simulink model "SST_FINAL_SIMULINK"  (R2017b)
settings: Solver=ode14x  StartTime=0.0  StopTime=120/60  MaxStep=1e-4  RelTol=1e-3
values from neighbouring files (symbols this model uses):
  C_3P4L = (Potencia_nominal)/(2*pi*60*0.1*((Entrada)^2))    (= 0.00858724363662)    [SST_FINAL.m]
  C_HB = 50000/(0.6*60*pi*(11397^2))    (= 3.40358447746e-06)    [SST_FINAL.m]
  ca = 1/(L*a)    [SST_FINAL.m]
  CDAB1 = 50*(Pnom/3)/(Vmin_DAB1^2*Fsw_DAB)    [SST_FINAL.m]
  CDAB2 = 50*(Pnom/3)/(Vmin_DAB2^2*Fsw_DAB)    [SST_FINAL.m]
  E = Nm*Vout_HB    (= 11397)    [SST_FINAL.m]
  Fsw_DAB = 30e3    (= 30000)    [SST_FINAL.m]
  Fsw_HB = 15e3    (= 15000)    [SST_FINAL.m]
  Fsw_NPC = 5040    [SST_FINAL.m]
  Inom_HB = (50e3/(13200*sqrt(3)))*sqrt(2)    [SST_FINAL.m]
  Kc_I = H_infI    [SST_FINAL.m]
  Kc_V = H_infV    [SST_FINAL.m]
  KcI_DAB = H_infI_DAB    [SST_FINAL.m]
  KcV_DAB = H_infV_DAB    [SST_FINAL.m]
  Ki = 2.5641    [SST_FINAL.m]
  Kp = 0.00138    [SST_FINAL.m]
  L = ((0.03*Entrada))/((2*pi*60)*(Imax))    [SST_FINAL.m]
  L_DAB = (1/Ntr)*VDAB1*VDAB2*D*(1-D)/(2*Fsw_DAB*(Pnom/3))    (= 2.89591875e-05)    [SST_FINAL.m]
  L_HB = 50e-3    (= 0.05)    [SST_FINAL.m]
  m = (2*Voltaje_pico)/Entrada    [SST_FINAL.m]
  Pnom = 50e3    (= 50000)    [SST_FINAL.m]
  R_DAB = 30e3*2*pi*L_DAB*0.1    (= 0.545867824224)    [SST_FINAL.m]
  R_HB = 120*pi*L_HB*0.05    (= 0.942477796077)    [SST_FINAL.m]
  R_LOAD2 = VDAB2^2/(Pnom/3)    (= 9.26694)    [SST_FINAL.m]
  tauI_I = 1/(2*pi*F_lagI)    (= 0.00265258238486)    [SST_FINAL.m]
  tauI_V = 1/(2*pi*F_LagV)    (= 0.00039788735773)    [SST_FINAL.m]
  tauII_DAB = 1/(2*pi*F_lagI_DAB)    (= 0.00265258238486)    [SST_FINAL.m]
  tauIV_DAB = 1/(2*pi*F_lagV_DAB)    (= 0.265258238486)    [SST_FINAL.m]
  Ts = 1/(200*Fsw_DAB)    (= 1.66666666667e-07)    [SST_FINAL.m]
  uLmt_dDAB = 0.5    [SST_FINAL.m]
  uLmt_I = 0.05    [SST_FINAL.m]
  uLmt_V = Inom_HB    [SST_FINAL.m]
  VDAB1 = 11397    [SST_FINAL.m]
  VDAB2 = 393    [SST_FINAL.m]
  Vp = Entrada/2    (= 196.5)    [SST_FINAL.m]
  W = 120*pi    (= 376.991118431)    [SST_FINAL.m]
  w = 120*pi    (= 376.991118431)    [SST_FINAL.m]
libraries: powerlib x102, powerlib_meascontrol x26, simulink x16, dspstat3 x3
(part 1 of 2)
settings Model: SimulationMode=accelerator  Creator=Sergio  LastModifiedBy=Sergio

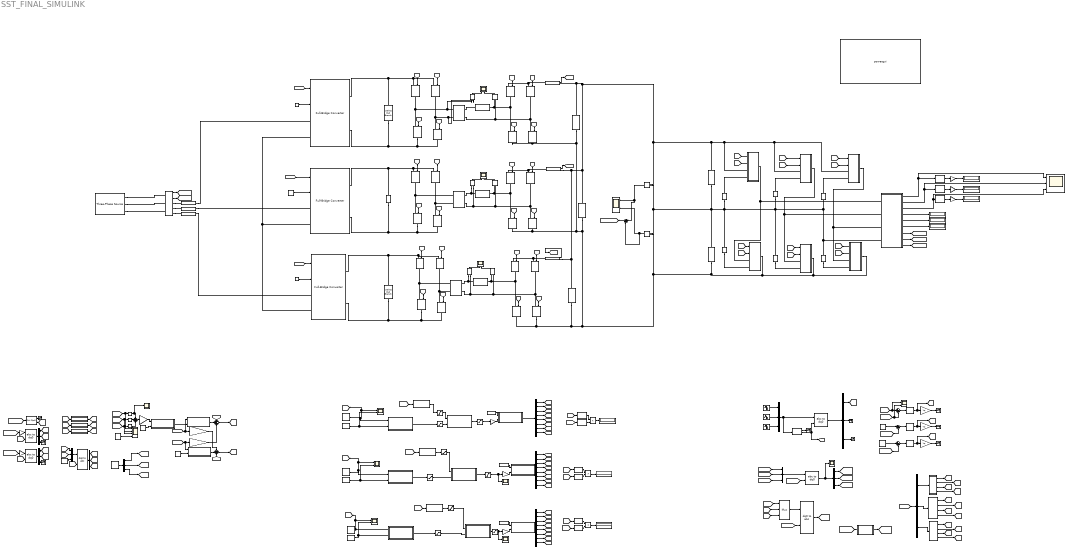
== system SST_FINAL_SIMULINK ==
  note: Fuente Trifásica Balanceada
      | Sec(+) Vnom=13.2 [kV]
  note: Medición de tensión y corriente
      | en media tensión
  note: Lazo de control de corriente
      | para etapa rectificadora
  note: Lazo de control de tensión
      | para etapa rectificadora
  note: Conversión de referencia abc a dq0
  note: Generación de pulsos - Metodo SPWM
  note: Conversión de referencia dq0 a abc
  note: Transformador Trifásico de Estado Sólido de Flujo Unidireccional de tres etapas de 13.2KV a 220V
  note: CONTROLADOR Y MODULADOR ETAPA AC-DC
  note: CONTROLADOR Y MODULADOR ETAPA DC-DC
  note: MODULADOR PSM
  note: MODULADOR PSM
  note: MODULADOR PSM
  note: CONTROLADOR LAZO
      | DE CORRIENTE
  note: CONTROLADOR LAZO
      | DE CORRIENTE
  note: CONTROLADOR LAZO
      | DE CORRIENTE
  note: CONTROLADOR LAZO
      | DE TENSIÓN
  note: CONTROLADOR LAZO
      | DE TENSIÓN
  note: CONTROLADOR LAZO
      | DE TENSIÓN
  note: POTENCIA DAB1
  note: POTENCIA DAB2
  note: POTENCIA DAB3
  note: CONTROLADOR Y MODULADOR ETAPA DC-AC
  note: ETAPA AC-DC
  note: ETAPA DC-DC
  note: ETAPA DC-AC
  note: CARGA CONECTADA EN Y
  note: TENSIONES DE LINEA EN LA CARGA
  note: TENSIONES RMS DE LINEA EN LA CARGA
  note: THD VAB
  note: THD VBC
  note: THD VCA
  note: TENSIONES CHB
  note: TENSIONES CHB
      | AVERAGE
  note: TENSIÓN VDAB2
  note: TENSIÓN VDAB2
  note: TENSIÓN VDAB2
  note: TENSIONES FASE DE REFERENCIA EN DQ0
  note: TENSIONES FASE MEDIDAS EN DQ0
  note: BALANCEO DE LAS CAPACITANCIAS NPC
  note: CONTROLADOR DE TENSIÓN EN EL DOMINIO DQ0
  note: CONVERSIÓN DE DQ0 A ABC DE LOS PULSOS
  note: GENERACIÓN DE PULSOS METODO SPWM
  note: TENSIÓN CAPACITANCIAS NPC
  CONTROL_ID_buck2 : MATLAB Function  TreatAsAtomicUnit=on
  CONTROL_ID_buck3 : MATLAB Function  TreatAsAtomicUnit=on
  CONTROL_ID_buck5 : MATLAB Function  TreatAsAtomicUnit=on
  CONTROL_ID_buck6 : MATLAB Function  TreatAsAtomicUnit=on
  CONTROL_ID_buck8 : MATLAB Function  TreatAsAtomicUnit=on
  CONTROL_ID_buck9 : MATLAB Function  TreatAsAtomicUnit=on
  Carga R con Filtro LC : Subsystem
  Constant : Constant  Value=VDAB2  SampleTime=Ts
  Constant{3..5,10,12,19..20} (7 alike) : Constant  Value=0
  Constant11 : Constant
  Constant8 : Constant  Value=VDAB2  SampleTime=Ts
  Constant9 : Constant  Value=VDAB2  SampleTime=Ts
  Current Measurement1 : powerlib/Measurements/Current Measurement  PhasorSimulation=off  OutputType=Complex  PSBequivalent=0
  Current Measurement2 : powerlib/Measurements/Current Measurement  PhasorSimulation=off  OutputType=Complex  PSBequivalent=0
  Current Measurement3 : powerlib/Measurements/Current Measurement  PhasorSimulation=off  OutputType=Complex  PSBequivalent=0
  D{1..5,7} (6 alike) : powerlib/Power Electronics/Diode  Ron=0.001  Lon=0  Vf=0  IC=0  UseSnubber=off  Rs=500  Cs=250e-9  Measurements=off
  DAB1_S{1..24} (24 alike) : powerlib/Power Electronics/IGBT//Diode  Ron=1e-3  Rs=1e5  Cs=inf  Measurements=off
  Demux : Demux  Outputs=8
  Demux1 : Demux  Outputs=8
  Demux{7..13} (7 alike) : Demux  Outputs=3
  Demux2 : Demux  Outputs=8
  Display{2..4,7..12} (9 alike) : Display
  Fase A1 : Sin  Amplitude=(220*sqrt(2))/sqrt(3)  Frequency=120*pi  SampleTime=0
  Fase B1 : Sin  Amplitude=(220*sqrt(2))/sqrt(3)  Frequency=120*pi  Phase=-120*pi/180  SampleTime=0
  Fase C1 : Sin  Amplitude=(220*sqrt(2))/sqrt(3)  Frequency=120*pi  Phase=120*pi/180  SampleTime=0
  Gain10 : Gain  Gain=100
  Gain11 : Gain  Gain=Vp
  Gain12 : Gain  Gain=Vp
  Gain13 : Gain  Gain=Vp
  Gain14 : Gain  Gain=1/E
  Gain15 : Gain  Gain=1/Inom_HB
  Gain16 : Gain  Gain=1/(3*E)
  Gain17 : Gain  Gain=W*L_HB*Inom_HB/E
  Gain18 : Gain  Gain=W*L_HB*Inom_HB/E
  Gain2 : Gain  Gain=pi
  Gain3 : Gain  Gain=100
  Gain4 : Gain  Gain=pi
  Gain5 : Gain  Gain=pi
  Gain8 : Gain  Gain=100
  H-Bridge A : powerlib/Power Electronics/Full-Bridge Converter  ModelType=Switching devices  Ron=1e-3  Rs=1e6  Cs=inf  Vforward=[0,0]  Ron_Diode=1e-3  Rs_Diode=1e6  Cs_Diode=inf  Vf_Diode=1e-3  Rs_CurrentSource=inf
      settings: SourceProductName=Simscape Power Systems  SourceProductBaseCode=PS
  H-Bridge B : powerlib/Power Electronics/Full-Bridge Converter  ModelType=Switching devices  Ron=1e-3  Rs=1e6  Cs=inf  Vforward=[0,0]  Ron_Diode=1e-3  Rs_Diode=1e6  Cs_Diode=inf  Vf_Diode=1e-3  Rs_CurrentSource=inf
      settings: SourceProductName=Simscape Power Systems  SourceProductBaseCode=PS
  H-Bridge C : powerlib/Power Electronics/Full-Bridge Converter  ModelType=Switching devices  Ron=1e-3  Rs=1e6  Cs=inf  Vforward=[0,0]  Ron_Diode=1e-3  Rs_Diode=1e6  Cs_Diode=inf  Vf_Diode=1e-3  Rs_CurrentSource=inf
      settings: SourceProductName=Simscape Power Systems  SourceProductBaseCode=PS
  LA : powerlib/Elements/Series RLC Branch  LConnTagsString=__new0  RConnTagsString=__new0  BranchType=RL  Resistance=R_HB  Inductance=L_HB  SetiL0=off  InitialCurrent=Inom  Capacitance=1e-6  Setx0=off  InitialVoltage=0  Measurements=None
  LB : powerlib/Elements/Series RLC Branch  LConnTagsString=__new0  RConnTagsString=__new0  BranchType=RL  Resistance=R_HB  Inductance=L_HB  SetiL0=off  InitialCurrent=Inom  Capacitance=1e-6  Setx0=off  InitialVoltage=0  Measurements=None
  LC : powerlib/Elements/Series RLC Branch  LConnTagsString=__new0  RConnTagsString=__new0  BranchType=RL  Resistance=R_HB  Inductance=L_HB  SetiL0=off  InitialCurrent=Inom  Capacitance=1e-6  Setx0=off  InitialVoltage=0  Measurements=None
  Linear Transformer1 : powerlib/Elements/Linear Transformer  UNITS=pu  NominalPower=[Pnom Fsw_DAB]  winding1=[VDAB1 0 0]  winding2=[VDAB2 0 0]  ThreeWindings=off  winding3=[ 315e3 0.002 0.08 ]  RmLm=[100e6 inf]  Measurements=None  DataType=off
  Linear Transformer2 : powerlib/Elements/Linear Transformer  UNITS=pu  NominalPower=[Pnom Fsw_DAB]  winding1=[VDAB1 0 0]  winding2=[VDAB2 0 0]  ThreeWindings=off  winding3=[ 315e3 0.002 0.08 ]  RmLm=[100e6 inf]  Measurements=None  DataType=off
  Linear Transformer3 : powerlib/Elements/Linear Transformer  UNITS=pu  NominalPower=[Pnom Fsw_DAB]  winding1=[VDAB1 0 0]  winding2=[VDAB2 0 0]  ThreeWindings=off  winding3=[ 315e3 0.002 0.08 ]  RmLm=[100e6 inf]  Measurements=None  DataType=off
  MATLAB Function2 : MATLAB Function  TreatAsAtomicUnit=on
  MATLAB Function3 : MATLAB Function  TreatAsAtomicUnit=on
  MATLAB Function4 : MATLAB Function  TreatAsAtomicUnit=on
  MATLAB Function5 : MATLAB Function  TreatAsAtomicUnit=on
  MATLAB Function6 : MATLAB Function  TreatAsAtomicUnit=on
  MATLAB Function7 : MATLAB Function  TreatAsAtomicUnit=on
  Mean{,1..5} (6 alike) : powerlib_meascontrol/Measurements/Mean  Freq=Fsw_DAB  Vinit=0  Ts=Ts
  Mean6 : powerlib_meascontrol/Measurements/Mean  Freq=120  Vinit=0  Ts=Ts
  Mean7 : powerlib_meascontrol/Measurements/Mean  Freq=120  Vinit=0  Ts=Ts
  Mean8 : powerlib_meascontrol/Measurements/Mean  Freq=120  Vinit=0  Ts=Ts
  Moving Average : dspstat3/Moving Average  Method=Sliding window  SpecifyWindowLength=on  WindowLength=1000  ForgettingFactor=0.9  SimulateUsing=Code generation
  Moving Average1 : dspstat3/Moving Average  Method=Sliding window  SpecifyWindowLength=on  WindowLength=1000  ForgettingFactor=0.9  SimulateUsing=Code generation
  Moving Average2 : dspstat3/Moving Average  Method=Sliding window  SpecifyWindowLength=on  WindowLength=1000  ForgettingFactor=0.9  SimulateUsing=Code generation
  Multimeter : powerlib/Measurements/Multimeter  PhasorSimulation=off  OutputType=Complex  sel=3  L=6  Gain=1  yselected={'Ub: Series RLC Branch16'};  PSBOutputType=1  PSBequivalent=0  AxesSetting=[0,0.1,-100,100]  Display=0  SavedBlockNames=-11
  Multimeter1 : powerlib/Measurements/Multimeter  PhasorSimulation=off  OutputType=Complex  sel=1  L=6  Gain=1  yselected={'Ub: Series RLC Branch13'};  PSBOutputType=1  PSBequivalent=0  AxesSetting=[0,0.1,-100,100]  Display=0  SavedBlockNames=-11
  Multimeter2 : powerlib/Measurements/Multimeter  PhasorSimulation=off  OutputType=Complex  sel=2  L=6  Gain=1  yselected={'Ub: Series RLC Branch14'};  PSBOutputType=1  PSBequivalent=0  AxesSetting=[0,0.1,-100,100]  Display=0  SavedBlockNames=-11
  Multimeter4 : powerlib/Measurements/Multimeter  PhasorSimulation=off  OutputType=Complex  sel=[4 5 6]  L=6  Gain=[1 1 1]  yselected={'Ub: Vout_HBa','Ub: Vout_HBb','Ub: Vout_HBc'};  PSBOutputType=1  PSBequivalent=0  AxesSetting=[0,0.1,-100,100]  Display=0  SavedBlockNames=-11
  Mux{,2..3,5} (4 alike) : Mux  Inputs=3
  PID Controller1 : simulink/Continuous/PID Controller  Controller=PI  TimeDomain=Continuous-time  SampleTime=-1  IntegratorMethod=Forward Euler  FilterMethod=Forward Euler  Form=Parallel  UseFilter=on  ControllerParametersSource=internal  P=Kp  I=Ki  D=0.00026179  N=100  InitialConditionSource=internal  InitialConditionForIntegrator=0  InitialConditionForFilter=0  ExternalReset=none  LimitOutput=off  UpperSaturationLimit=inf  LowerSaturationLimit=-inf  LinearizeAsGain=on  AntiWindupMode=none  Kb=1  TrackingMode=off  Kt=1  PParamMin=[]  PParamMax=[]  IParamMin=[]  IParamMax=[]  DParamMin=[]  DParamMax=[]  NParamMin=[]  NParamMax=[]  KbParamMin=[]  KbParamMax=[]  KtParamMin=[]  KtParamMax=[]  POutMin=[]  POutMax=[]  IOutMin=[]  IOutMax=[]  DOutMin=[]  DOutMax=[]  NOutMin=[]  NOutMax=[]  KbOutMin=[]  KbOutMax=[]  KtOutMin=[]  KtOutMax=[]  IntegratorOutMin=[]  IntegratorOutMax=[]  FilterOutMin=[]  FilterOutMax=[]  SumOutMin=[]  SumOutMax=[]  SumI1OutMin=[]  SumI1OutMax=[]  SumI2OutMin=[]  SumI2OutMax=[]  SumI3OutMin=[]  SumI3OutMax=[]  SumDOutMin=[]  SumDOutMax=[]  SaturationOutMin=[]  SaturationOutMax=[]  IntegratorContinuousStateAttributes=''  IntegratorStateMustResolveToSignalObject=off  IntegratorRTWStateStorageClass=Auto  FilterContinuousStateAttributes=''  FilterStateMustResolveToSignalObject=off  FilterRTWStateStorageClass=Auto  DifferentiatorICPrevScaledInput=0  DifferentiatorOutMin=[]  DifferentiatorOutMax=[]  InitialConditionSetting=State (most efficient)  FilterDiffOutCoefMin=[]  FilterDiffOutCoefMax=[]  SumDenOutMin=[]  SumDenOutMax=[]  SumNumOutMin=[]  SumNumOutMax=[]  ReciprocalOutMin=[]  ReciprocalOutMax=[]  DivideOutMin=[]  DivideOutMax=[]  TunerSelectOption=Transfer Function Based (PID Tuner App)
  PID Controller2 : simulink/Continuous/PID Controller  Controller=PI  TimeDomain=Continuous-time  SampleTime=-1  IntegratorMethod=Forward Euler  FilterMethod=Forward Euler  Form=Parallel  UseFilter=on  ControllerParametersSource=internal  P=Kp  I=Ki  D=0.00026179  N=100  InitialConditionSource=internal  InitialConditionForIntegrator=0  InitialConditionForFilter=0  ExternalReset=none  LimitOutput=off  UpperSaturationLimit=inf  LowerSaturationLimit=-inf  LinearizeAsGain=on  AntiWindupMode=none  Kb=1  TrackingMode=off  Kt=1  PParamMin=[]  PParamMax=[]  IParamMin=[]  IParamMax=[]  DParamMin=[]  DParamMax=[]  NParamMin=[]  NParamMax=[]  KbParamMin=[]  KbParamMax=[]  KtParamMin=[]  KtParamMax=[]  POutMin=[]  POutMax=[]  IOutMin=[]  IOutMax=[]  DOutMin=[]  DOutMax=[]  NOutMin=[]  NOutMax=[]  KbOutMin=[]  KbOutMax=[]  KtOutMin=[]  KtOutMax=[]  IntegratorOutMin=[]  IntegratorOutMax=[]  FilterOutMin=[]  FilterOutMax=[]  SumOutMin=[]  SumOutMax=[]  SumI1OutMin=[]  SumI1OutMax=[]  SumI2OutMin=[]  SumI2OutMax=[]  SumI3OutMin=[]  SumI3OutMax=[]  SumDOutMin=[]  SumDOutMax=[]  SaturationOutMin=[]  SaturationOutMax=[]  IntegratorContinuousStateAttributes=''  IntegratorStateMustResolveToSignalObject=off  IntegratorRTWStateStorageClass=Auto  FilterContinuousStateAttributes=''  FilterStateMustResolveToSignalObject=off  FilterRTWStateStorageClass=Auto  DifferentiatorICPrevScaledInput=0  DifferentiatorOutMin=[]  DifferentiatorOutMax=[]  InitialConditionSetting=State (most efficient)  FilterDiffOutCoefMin=[]  FilterDiffOutCoefMax=[]  SumDenOutMin=[]  SumDenOutMax=[]  SumNumOutMin=[]  SumNumOutMax=[]  ReciprocalOutMin=[]  ReciprocalOutMax=[]  DivideOutMin=[]  DivideOutMax=[]  TunerSelectOption=Transfer Function Based (PID Tuner App)
  PID Controller7 : simulink/Continuous/PID Controller  Controller=PI  TimeDomain=Continuous-time  SampleTime=-1  IntegratorMethod=Forward Euler  FilterMethod=Forward Euler  Form=Parallel  UseFilter=on  ControllerParametersSource=internal  P=Kp  I=Ki  D=0.00026179  N=100  InitialConditionSource=internal  InitialConditionForIntegrator=0  InitialConditionForFilter=0  ExternalReset=none  LimitOutput=off  UpperSaturationLimit=inf  LowerSaturationLimit=-inf  LinearizeAsGain=on  AntiWindupMode=none  Kb=1  TrackingMode=off  Kt=1  PParamMin=[]  PParamMax=[]  IParamMin=[]  IParamMax=[]  DParamMin=[]  DParamMax=[]  NParamMin=[]  NParamMax=[]  KbParamMin=[]  KbParamMax=[]  KtParamMin=[]  KtParamMax=[]  POutMin=[]  POutMax=[]  IOutMin=[]  IOutMax=[]  DOutMin=[]  DOutMax=[]  NOutMin=[]  NOutMax=[]  KbOutMin=[]  KbOutMax=[]  KtOutMin=[]  KtOutMax=[]  IntegratorOutMin=[]  IntegratorOutMax=[]  FilterOutMin=[]  FilterOutMax=[]  SumOutMin=[]  SumOutMax=[]  SumI1OutMin=[]  SumI1OutMax=[]  SumI2OutMin=[]  SumI2OutMax=[]  SumI3OutMin=[]  SumI3OutMax=[]  SumDOutMin=[]  SumDOutMax=[]  SaturationOutMin=[]  SaturationOutMax=[]  IntegratorContinuousStateAttributes=''  IntegratorStateMustResolveToSignalObject=off  IntegratorRTWStateStorageClass=Auto  FilterContinuousStateAttributes=''  FilterStateMustResolveToSignalObject=off  FilterRTWStateStorageClass=Auto  DifferentiatorICPrevScaledInput=0  DifferentiatorOutMin=[]  DifferentiatorOutMax=[]  InitialConditionSetting=State (most efficient)  FilterDiffOutCoefMin=[]  FilterDiffOutCoefMax=[]  SumDenOutMin=[]  SumDenOutMax=[]  SumNumOutMin=[]  SumNumOutMax=[]  ReciprocalOutMin=[]  ReciprocalOutMax=[]  DivideOutMin=[]  DivideOutMax=[]  TunerSelectOption=Transfer Function Based (PID Tuner App)
  PLL (3ph)1 : powerlib_meascontrol/PLL/PLL (3ph)  Fmin=45  Par_Init=[0, 60]  ParK=[180, 3200, 1]  TcD=1e-4  MaxRateChangeFreq=12  FilterCutOffFreq=25  Ts=Ts  AGC=on
  PLL (3ph)2 : powerlib_meascontrol/PLL/PLL (3ph)  Fmin=45  Par_Init=[0, 60]  ParK=[180, 3200, 1]  TcD=1e-4  MaxRateChangeFreq=12  FilterCutOffFreq=25  Ts=Ts  AGC=on
  Portadora : simulink/Sources/Repeating Sequence  rep_seq_t=[0 1]/Fsw_DAB  rep_seq_y=[0 2*pi]
  Portadora1 : simulink/Sources/Repeating Sequence  rep_seq_t=[0 1]/Fsw_DAB  rep_seq_y=[0 2*pi]
  Portadora2 : simulink/Sources/Repeating Sequence  rep_seq_t=[0 1]/Fsw_DAB  rep_seq_y=[0 2*pi]
  Product1 : Product
  Product2 : Product
  Product3 : Product
  Saturation : Saturate
  Saturation{4,7,10..12} (5 alike) : Saturate  UpperLimit=5*VDAB2/R_LOAD2  LowerLimit=0
  Saturation5 : Saturate
  Saturation8 : Saturate
  Saturation9 : Saturate  UpperLimit=2*VDAB2/R_LOAD2  LowerLimit=0
  Scope{,3..6,9..10,16} (8 alike) : Scope  NumInputPorts=2
  Scope{7,11,18,21} (4 alike) : Scope
  Scope14 : Scope  NumInputPorts=4
  Scope15 : Scope  NumInputPorts=3
  Series RLC Branch : powerlib/Elements/Series RLC Branch  LConnTagsString=__new0  RConnTagsString=__new0  BranchType=RC  Resistance=0.0001  Inductance=1e-3  SetiL0=off  InitialCurrent=0  Capacitance=2*C_3P4L  Setx0=on  InitialVoltage=VDAB2/2  Measurements=None
  Series RLC Branch13 : powerlib/Elements/Series RLC Branch  LConnTagsString=__new0  RConnTagsString=__new0  BranchType=C  Resistance=1  Inductance=1e-3  SetiL0=off  InitialCurrent=0  Capacitance=CDAB2  Setx0=off  InitialVoltage=VDAB2  Measurements=Branch voltage
  Series RLC Branch14 : powerlib/Elements/Series RLC Branch  LConnTagsString=__new0  RConnTagsString=__new0  BranchType=C  Resistance=1  Inductance=1e-3  SetiL0=off  InitialCurrent=0  Capacitance=CDAB2  Setx0=off  InitialVoltage=VDAB2  Measurements=Branch voltage
  Series RLC Branch16 : powerlib/Elements/Series RLC Branch  LConnTagsString=__new0  RConnTagsString=__new0  BranchType=C  Resistance=1  Inductance=1e-3  SetiL0=off  InitialCurrent=0  Capacitance=CDAB2  Setx0=off  InitialVoltage=VDAB2  Measurements=Branch voltage
  Series RLC Branch18 : powerlib/Elements/Series RLC Branch  LConnTagsString=__new0  RConnTagsString=__new0  BranchType=RL  Resistance=R_DAB  Inductance=L_DAB  SetiL0=off  InitialCurrent=0  Capacitance=1e-6  Setx0=off  InitialVoltage=0  Measurements=None
  Series RLC Branch19 : powerlib/Elements/Series RLC Branch  LConnTagsString=__new0  RConnTagsString=__new0  BranchType=RL  Resistance=R_DAB  Inductance=L_DAB  SetiL0=off  InitialCurrent=0  Capacitance=1e-6  Setx0=off  InitialVoltage=0  Measurements=None
  Series RLC Branch20 : powerlib/Elements/Series RLC Branch  LConnTagsString=__new0  RConnTagsString=__new0  BranchType=RL  Resistance=R_DAB  Inductance=L_DAB  SetiL0=off  InitialCurrent=0  Capacitance=1e-6  Setx0=off  InitialVoltage=0  Measurements=None
  Series RLC Branch7 : powerlib/Elements/Series RLC Branch  LConnTagsString=__new0  RConnTagsString=__new0  BranchType=RC  Resistance=0.0001  Inductance=1e-3  SetiL0=off  InitialCurrent=0  Capacitance=2*C_3P4L  Setx0=on  InitialVoltage=VDAB2/2  Measurements=None
  Subsystem : Subsystem
  Subsystem1 : Subsystem
  Subsystem10 : Subsystem
  Subsystem11 : Subsystem
  Subsystem12 : Subsystem
  Subsystem2 : Subsystem
  Subsystem3 : Subsystem
  Subsystem4 : Subsystem
  Subsystem5 : Subsystem
  Subsystem6 : Subsystem
  Subsystem7 : Subsystem
  Subsystem8 : Subsystem
  Subsystem9 : Subsystem
  Sum10 : Sum  Inputs=+-+
  Sum12 : Sum  Inputs=--+
  Sum13 : Sum  Inputs=+++
  Sum{3..4,6..7} (4 alike) : Sum  Inputs=|+-
  THD4 : powerlib_meascontrol/Measurements/THD  Freq=60  Ts=0
  THD5 : powerlib_meascontrol/Measurements/THD  Freq=60  Ts=0
  THD6 : powerlib_meascontrol/Measurements/THD  Freq=60  Ts=0
  Terminator{3..11} (9 alike) : Terminator
  Three-Phase V-I Measurement : powerlib/Measurements/Three-Phase V-I Measurement  VoltageMeasurement=phase-to-ground  SetLabelV=off  LabelV=Vabc  Vpu=off  VpuLL=off  CurrentMeasurement=yes  SetLabelI=off  LabelI=Iabc  Ipu=off  Pbase=100e6  Vbase=500e3  OutputType=Complex  PhasorSimulation=off  PSBequivalent=0
  Three-Phase Source : powerlib/Electrical Sources/Three-Phase Source  InternalConnection=Yg  VoltagePhases=off  Voltage=13200  PhaseAngle=0  Voltage_phases=[25e3 25e3 25e3]/sqrt(3)  PhaseAngles_phases=[0 -120 +120]  Frequency=60  NonIdealSource=off  SpecifyImpedance=off  Resistance=0.8929  Inductance=16.58e-3  ShortCircuitLevel=100e6  BaseVoltage=25e3  XRratio=7  BusType=swing  Pref=50e3  Qref=0  Prefabc=[10e3, 10e3, 10e3]  Qrefabc=[0, 0, 0]  Qmin=-inf  Qmax=inf
  Voltage Measurement{,1..7} (8 alike) : powerlib/Measurements/Voltage Measurement  PhasorSimulation=off  OutputType=Complex  PSBequivalent=0
  Vout_HBa : powerlib/Elements/Series RLC Branch  LConnTagsString=__new0  RConnTagsString=__new0  BranchType=C  Resistance=1  Inductance=1e-3  SetiL0=off  InitialCurrent=0  Capacitance=(C_HB+CDAB1)  Setx0=on  InitialVoltage=Vout_HB  Measurements=Branch voltage
  Vout_HBb : powerlib/Elements/Series RLC Branch  LConnTagsString=__new0  RConnTagsString=__new0  BranchType=C  Resistance=1  Inductance=1e-3  SetiL0=off  InitialCurrent=0  Capacitance=(C_HB+CDAB1)  Setx0=on  InitialVoltage=Vout_HB  Measurements=Branch voltage
  Vout_HBc : powerlib/Elements/Series RLC Branch  LConnTagsString=__new0  RConnTagsString=__new0  BranchType=C  Resistance=1  Inductance=1e-3  SetiL0=off  InitialCurrent=0  Capacitance=(C_HB+CDAB1)  Setx0=on  InitialVoltage=Vout_HB  Measurements=Branch voltage
  Vout_máx : Constant  Value=E  SampleTime=Ts
  abc to dq{2..5} (4 alike) : powerlib_meascontrol/Transformations/abc to dq0  Alignment=90 degrees behind phase A axis
  dq0 to abc2 : powerlib_meascontrol/Transformations/dq0 to abc  Alignment=90 degrees behind phase A axis
  dq0 to abc3 : powerlib_meascontrol/Transformations/dq0 to abc  Alignment=90 degrees behind phase A axis
  powergui1 : powerlib/powergui  Priority=1  SimulationMode=Discrete  SampleTime=Ts  frequency=60  Iterations=50  frequencyindice=60  Pbase=100e6  ErrMax=1e-4  UnitsV=kV  UnitsW=MW  buscounter=0  FunctionMessages=off  echomessages=off  EnableUseOfTLC=off  CurrentSourceSwitches=off  DisableSnubberDevices=off  DisableRonSwitches=off  DisableVfSwitches=off  DisplayEquations=off  SolverType=Tustin/Backward Euler (TBE)  Interpol=off  ExternalGateDelay=off  methode=off  Ts=100  x0status=blocks  SPID=on  SwTol=0  HookPort=off  RestoreLinks=warning  ResistiveCurrentMeasurement=off  Frange=[0:2:500]  Ylog=off  Xlog=on  ShowGrid=off  save=off  variable=ZData  structure=0  ZoomFFT=off  StartTime=0.0  cycles=1  DisplayStyle=1  fundamental=60  FreqAxis=off  MaxFrequency=1000  frequencyindicesteady=1  RmsSteady=1  display=off
  tag scope: Corrientes_MV=global, D01=global, Dd1=global, Dq1=global, IDAB2A=global, IDAB2B=global, IDAB2C=global, Pulsos_abc=global, S10=global, S11=global, S12=global, S13=global, S14=global, S15=global, S16=global, S17=global, S18=global, S19=global, S1=global, S20=global, S21=global, S22=global, S23=global, S24=global, S2=global, S3=global, S4=global, S5=global, S6=global, S7=global, S8=global, S9=global, Tensiones_MV=global, V0_measure=global, Va_measure=global, Vb_measure=global, Vc_measure=global, Vd_measure=global, Vd_ref=global, VdcA=global, VdcB=global, VdcC=global, Vq_measure=global, capacitores=global, offset=global, s11=global, s12=global, s13=global, s14=global, s21=global, s22=global, s23=global, s24=global, s31=global, s32=global, s33=global, s34=global, wt=global
  wires:
  [Sb_HB] -> H-Bridge B/1
  Constant5/1 -> H-Bridge C/2
  [Sc_HB] -> H-Bridge A/1
  [Sa_HB] -> H-Bridge C/1
  Constant4/1 -> H-Bridge B/2
  Three-Phase V-I Measurement/2 -> [Corrientes_MV]
  Constant3/1 -> H-Bridge A/2
  Three-Phase V-I Measurement/1 -> [Tensiones_MV]
  [S4] -> DAB1_S12/1
  Demux1/4 -> [S12]
  Demux2/3 -> [S19]
  Saturation8/1 -> Scope11/1, Gain5/1
  Current Measurement1/1 -> [IDAB2B]
  CONTROL_ID_buck9/1(uCur) -> Saturation4/1
  [S5] -> DAB1_S13/1
  Current Measurement2/1 -> [IDAB2C]
  MATLAB Function2/1(S_dab) -> Demux/1
  Current Measurement3/1 -> [IDAB2A]
  CONTROL_ID_buck3/1(uCur) -> Saturation9/1
  Mean3/1 -> Product2/2
  Demux2/5 -> [S21]
  CONTROL_ID_buck5/1(uCur) -> Saturation/1
  CONTROL_ID_buck6/1(uCur) -> Saturation5/1
  [IDAB2C] -> Moving Average2/1
  Demux1/5 -> [S13]
  Moving Average2/1 -> Saturation11/1
  [IDAB2B] -> Moving Average1/1
  [S19] -> DAB1_S19/1
  Saturation4/1 -> CONTROL_ID_buck5/2(rCur)
  Demux/1 -> [S1]
  Saturation7/1 -> CONTROL_ID_buck6/2(rCur)
  [IDAB2C] -> Mean5/1
  Gain4/1 -> MATLAB Function3/2(d_dab)
  Moving Average1/1 -> Saturation12/1
  Demux/3 -> [S3]
  Product3/1 -> Display9/1
  CONTROL_ID_buck8/1(uCur) -> Saturation8/1
  [S24] -> DAB1_S24/1
  Saturation10/1 -> CONTROL_ID_buck5/1(yCur)
  Voltage Measurement3/1 -> Scope5/1
  Demux2/8 -> [S24]
  [IDAB2A] -> Moving Average/1
  Saturation12/1 -> CONTROL_ID_buck6/1(yCur)
  Voltage Measurement4/1 -> Scope5/2
  Demux/2 -> [S2]
  [S21] -> DAB1_S21/1
  [S23] -> DAB1_S23/1
  [S7] -> DAB1_S15/1
  Multimeter1/1 -> CONTROL_ID_buck2/1(yCur), Scope6/1, [VdcB]
  Voltage Measurement6/1 -> Scope9/2
  [VdcA] -> Mean/1
  [S22] -> DAB1_S22/1
  [IDAB2B] -> Mean3/1
  MATLAB Function4/1(S_dab) -> Demux2/1
  Product2/1 -> Display8/1
  MATLAB Function3/1(S_dab) -> Demux1/1
  [IDAB2A] -> Mean1/1
  Mean4/1 -> Product3/1
  Voltage Measurement5/1 -> Scope9/1
  [S10] -> DAB1_S2/1
  [S11] -> DAB1_S3/1
  Constant/1 -> CONTROL_ID_buck9/2(rCur), Scope4/2
  [S3] -> DAB1_S11/1
  [S15] -> DAB1_S7/1
  [S17] -> DAB1_S17/1
  Mean/1 -> Product1/1
  Demux/8 -> [S8]
  Demux2/4 -> [S20]
  [S12] -> DAB1_S4/1
  Demux1/1 -> [S9]
  Constant9/1 -> CONTROL_ID_buck3/2(rCur), Scope10/2
  Saturation9/1 -> CONTROL_ID_buck8/2(rCur)
  Moving Average/1 -> Saturation10/1
  Mean1/1 -> Product1/2
  [VdcB] -> Mean2/1
  Mean2/1 -> Product2/1
  Portadora/1 -> MATLAB Function2/1(Carrier_dab)
  Demux/7 -> [S7]
  Demux1/2 -> [S10]
  [S14] -> DAB1_S6/1
  Mean5/1 -> Product3/2
  [S1] -> DAB1_S9/1
  [S6] -> DAB1_S14/1
  CONTROL_ID_buck2/1(uCur) -> Saturation7/1
  Multimeter/1 -> CONTROL_ID_buck9/1(yCur), Scope4/1, [VdcA]
  Portadora2/1 -> MATLAB Function4/1(Carrier_dab)
  [S9] -> DAB1_S1/1
  Saturation5/1 -> Gain4/1, Scope7/1
  Demux2/6 -> [S22]
  [S8] -> DAB1_S16/1
  Multimeter2/1 -> CONTROL_ID_buck3/1(yCur), Scope10/1, [VdcC]
  Demux/6 -> [S6]
  Demux/4 -> [S4]
  Saturation11/1 -> CONTROL_ID_buck8/1(yCur)
  Portadora1/1 -> MATLAB Function3/1(Carrier_dab)
  Saturation/1 -> Gain2/1
  Demux/5 -> [S5]
  Demux2/1 -> [S17]
  Demux2/2 -> [S18]
  Constant8/1 -> CONTROL_ID_buck2/2(rCur), Scope6/2
  Voltage Measurement1/1 -> Scope3/1
  Voltage Measurement2/1 -> Scope3/2
  [S16] -> DAB1_S8/1
  Demux1/6 -> [S14]
  [VdcC] -> Mean4/1
  [S13] -> DAB1_S5/1
  Demux1/3 -> [S11]
  Product1/1 -> Display7/1
  Gain5/1 -> MATLAB Function4/2(d_dab)
  Demux2/7 -> [S23]
  Demux1/8 -> [S16]
  Demux1/7 -> [S15]
  [S2] -> DAB1_S10/1
  [S18] -> DAB1_S18/1
  [S20] -> DAB1_S20/1
  Gain2/1 -> MATLAB Function2/2(d_dab)
  Gain3/1 -> Display3/1
  THD5/1 -> Gain3/1
  Gain10/1 -> Display2/1
  THD4/1 -> Gain10/1
  THD6/1 -> Gain8/1
  Gain8/1 -> Display12/1
  Carga R con Filtro LC/2(Out2) -> Scope15/2, THD5/1
  Subsystem/1(Out1) -> [offset]
  [capacitores] -> Subsystem/1(In1)
  Carga R con Filtro LC/3(Out3) -> Scope15/3, THD6/1
  [s33] -> Subsystem10/1(In1)
  [s11] -> Subsystem1/1(In1)
  [s21] -> Subsystem7/1(In1)
  [s13] -> Subsystem5/1(In1)
  Sum7/1 -> [capacitores]
  [s32] -> Subsystem9/2(In2)
  [s22] -> Subsystem7/2(In2)
  [s12] -> Subsystem1/2(In2)
  [s23] -> Subsystem8/1(In1)
  [s24] -> Subsystem8/2(In2)
  [s34] -> Subsystem10/2(In2)
  Voltage Measurement7/1 -> Sum7/2, Scope/2
  [s31] -> Subsystem9/1(In1)
  Voltage Measurement/1 -> Sum7/1, Scope/1
  [s14] -> Subsystem5/2(In2)
  Carga R con Filtro LC/9(Out9) -> [Vc_measure]
  Carga R con Filtro LC/7(Out7) -> [Va_measure]
  Carga R con Filtro LC/8(Out8) -> [Vb_measure]
  Carga R con Filtro LC/6(Out6) -> Display11/1
  Carga R con Filtro LC/4(Out4) -> Display4/1
  Carga R con Filtro LC/5(Out5) -> Display10/1
  Carga R con Filtro LC/1(Out1) -> Scope15/1, THD4/1
  [Pulsos_abc] -> Demux8/1
  [Vd_ref] -> Scope16/1, Sum3/1
  [wt] -> dq0 to abc2/2
  dq0 to abc2/1 -> [Pulsos_abc]
  Demux7/2 -> [Vq_measure]
  [Dd1] -> Mux5/1
  PID Controller1/1 -> Gain11/1, [Dq1]
  [Vb_measure] -> Mux/2
  Demux9/2 -> Terminator4/1
  [D01] -> Mux5/3
  Fase A1/1 -> Mux3/1
  Sum4/1 -> PID Controller2/1
  Constant19/1 -> Sum6/1
  Sum3/1 -> PID Controller7/1
  Gain13/1 -> Terminator3/1
  Mux3/1 -> abc to dq3/1, PLL (3ph)1/1
  [Va_measure] -> Mux/1
  PLL (3ph)1/1 -> Terminator6/1
  Demux7/3 -> [V0_measure]
  Demux9/1 -> [Vd_ref]
  Fase B1/1 -> Mux3/2
  Mux/1 -> abc to dq2/1
  abc to dq2/1 -> Scope18/1, Demux7/1
  Gain11/1 -> Terminator5/1
  PID Controller7/1 -> [Dd1], Gain13/1
  [wt] -> abc to dq2/2
  Fase C1/1 -> Mux3/3
  Sum6/1 -> PID Controller1/1
  Mux5/1 -> dq0 to abc2/1
  PLL (3ph)1/2 -> [wt], abc to dq3/2
  Demux7/1 -> [Vd_measure]
  Demux9/3 -> Terminator7/1
  [Vc_measure] -> Mux/3
  [Dq1] -> Mux5/2
  abc to dq3/1 -> Demux9/1
  PID Controller2/1 -> Gain12/1, [D01]
  Gain12/1 -> Terminator8/1
  Constant20/1 -> Sum4/1
  Gain15/1 -> abc to dq5/1
  Sum13/1 -> Gain16/1
  Mean8/1 -> Sum13/3
  Mean6/1 -> Sum13/2
  Mean7/1 -> Scope21/1, Sum13/1
  Sum10/1 -> [Dd]
  Demux10/3 -> Terminator10/1
  Mux2/1 -> dq0 to abc3/1
  [DC_MT_A] -> Scope14/1, Mean7/1
  [Id_MV] -> MATLAB Function5/1(yCur), Gain17/1
  Demux13/1 -> [DC_MT_A]
  [db] -> Subsystem12/1(Referencia)
  Multimeter4/1 -> Demux13/1
  [DC_MT_B] -> Scope14/2, Mean6/1
  MATLAB Function7/1(uCur) -> MATLAB Function5/2(rCur)
  PLL (3ph)2/1 -> Terminator9/1
  Constant10/1 -> Mux2/3
  [Theta] -> abc to dq5/2
  Demux11/1 -> [Id_MV]
  MATLAB Function6/1(uCur) -> Sum12/2
  MATLAB Function5/1(uCur) -> Sum10/2
  Gain14/1 -> abc to dq4/1
  Demux12/2 -> [db]
  Gain18/1 -> Sum10/3
  [da] -> Subsystem4/1(Referencia)
  [Vd_MV] -> Sum10/1
  Demux10/1 -> [Vd_MV]
  Demux12/1 -> [da]
  Demux12/3 -> [dc]
  [Dq] -> Mux2/2
  Constant12/1 -> MATLAB Function6/2(rCur)
  [DC_MT_C] -> Scope14/3, Mean8/1
  Gain16/1 -> MATLAB Function7/1(yCur)
  Subsystem4/1(SW1) -> [Sa_HB]
  Demux11/2 -> [Iq_MV]
  [Corrientes_MV] -> Gain15/1
  Subsystem11/1(SW1) -> [Sc_HB]
  [Iq_MV] -> MATLAB Function6/1(yCur), Gain18/1
  [Theta] -> abc to dq4/2
  abc to dq5/1 -> Demux11/1
  Constant11/1 -> MATLAB Function7/2(rCur)
  Demux11/3 -> Terminator11/1
  Demux13/2 -> [DC_MT_B]
  Demux10/2 -> [Vq_MV]
  Gain17/1 -> Sum12/1
  [dc] -> Subsystem11/1(Referencia)
  [Tensiones_MV] -> Gain14/1
  [Dd] -> Mux2/1
  [Theta] -> dq0 to abc3/2
  [Tensiones_MV] -> PLL (3ph)2/1
  dq0 to abc3/1 -> Demux12/1
  PLL (3ph)2/2 -> [Theta]
  abc to dq4/1 -> Demux10/1
  Sum12/1 -> [Dq]
  [Vq_MV] -> Sum12/3
  Subsystem12/1(SW1) -> [Sb_HB]
  Demux13/3 -> [DC_MT_C]
  [Vq_measure] -> Sum6/2
  [V0_measure] -> Sum4/2
  [Vd_measure] -> Scope16/2, Sum3/2
  Vout_máx/1 -> Scope14/4
  Demux8/1 -> Subsystem2/1(In1)
  Subsystem2/1(Out1) -> [s11]
  Subsystem2/2(Out2) -> [s13]
  Subsystem2/3(Out3) -> [s14]
  Subsystem2/4(Out4) -> [s12]
  Demux8/2 -> Subsystem3/1(In1)
  Subsystem3/1(Out1) -> [s21]
  Subsystem3/2(Out2) -> [s23]
  Subsystem3/3(Out3) -> [s24]
  Subsystem3/4(Out4) -> [s22]
  Demux8/3 -> Subsystem6/1(In1)
  Subsystem6/1(Out1) -> [s31]
  Subsystem6/2(Out2) -> [s33]
  Subsystem6/3(Out3) -> [s34]
  Subsystem6/4(Out4) -> [s32]
  connections:
  Current Measurement2/RConn1 -- Series RLC Branch14/LConn1 -- Current Measurement1/RConn1 -- Series RLC Branch13/LConn1 -- Voltage Measurement/LConn1 -- Series RLC Branch/LConn1 -- Subsystem1/LConn1 -- Subsystem9/LConn1 -- Subsystem7/LConn1 -- Series RLC Branch16/LConn1 -- Current Measurement3/RConn1
  H-Bridge A/LConn2 -- H-Bridge C/LConn2 -- H-Bridge B/LConn2
  Three-Phase V-I Measurement/RConn2 -- LB/RConn1
  LC/LConn1 -- H-Bridge A/LConn1
  Three-Phase V-I Measurement/RConn3 -- LC/RConn1
  Three-Phase V-I Measurement/RConn1 -- LA/RConn1
  Three-Phase Source/RConn2 -- Three-Phase V-I Measurement/LConn2
  LB/LConn1 -- H-Bridge B/LConn1
  Three-Phase Source/RConn1 -- Three-Phase V-I Measurement/LConn1
  LA/LConn1 -- H-Bridge C/LConn1
  Three-Phase Source/RConn3 -- Three-Phase V-I Measurement/LConn3
  Voltage Measurement5/LConn2 -- Linear Transformer2/RConn2 -- DAB1_S24/LConn1 -- DAB1_S22/RConn1 -- Voltage Measurement6/LConn2
  Voltage Measurement4/LConn2 -- Linear Transformer3/RConn2 -- DAB1_S16/LConn1 -- DAB1_S14/RConn1
  Voltage Measurement6/LConn1 -- Series RLC Branch19/RConn1 -- DAB1_S23/LConn1 -- DAB1_S21/RConn1
  DAB1_S5/LConn1 -- DAB1_S6/LConn1 -- Current Measurement1/LConn1
  Voltage Measurement2/LConn2 -- Voltage Measurement1/LConn2 -- Linear Transformer1/RConn2 -- DAB1_S8/LConn1 -- DAB1_S6/RConn1
  DAB1_S22/LConn1 -- DAB1_S21/LConn1 -- Current Measurement2/LConn1
  Linear Transformer3/LConn2 -- Voltage Measurement3/LConn2 -- DAB1_S12/LConn1 -- DAB1_S10/RConn1
  Voltage Measurement5/LConn1 -- Linear Transformer2/RConn1 -- Series RLC Branch19/LConn1
  DAB1_S4/LConn1 -- Linear Transformer1/LConn2 -- DAB1_S2/RConn1
  DAB1_S3/LConn1 -- Linear Transformer1/LConn1 -- DAB1_S1/RConn1
  DAB1_S13/LConn1 -- DAB1_S14/LConn1 -- Current Measurement3/LConn1
  Linear Transformer2/LConn2 -- DAB1_S20/LConn1 -- DAB1_S18/RConn1
  Voltage Measurement4/LConn1 -- Series RLC Branch20/RConn1 -- DAB1_S15/LConn1 -- DAB1_S13/RConn1
  Linear Transformer1/RConn1 -- Voltage Measurement1/LConn1 -- Series RLC Branch18/LConn1
  Linear Transformer3/LConn1 -- Voltage Measurement3/LConn1 -- DAB1_S11/LConn1 -- DAB1_S9/RConn1
  Linear Transformer2/LConn1 -- DAB1_S19/LConn1 -- DAB1_S17/RConn1
  Voltage Measurement2/LConn1 -- Series RLC Branch18/RConn1 -- DAB1_S7/LConn1 -- DAB1_S5/RConn1
  Linear Transformer3/RConn1 -- Series RLC Branch20/LConn1
  DAB1_S17/LConn1 -- H-Bridge A/RConn1 -- Vout_HBa/LConn1 -- DAB1_S18/LConn1
  DAB1_S9/LConn1 -- Vout_HBc/LConn1 -- H-Bridge C/RConn1 -- DAB1_S10/LConn1
  DAB1_S11/RConn1 -- H-Bridge C/RConn2 -- Vout_HBc/RConn1 -- DAB1_S12/RConn1
  DAB1_S1/LConn1 -- H-Bridge B/RConn1 -- Vout_HBb/LConn1 -- DAB1_S2/LConn1
  DAB1_S3/RConn1 -- H-Bridge B/RConn2 -- Vout_HBb/RConn1 -- DAB1_S4/RConn1
  DAB1_S19/RConn1 -- H-Bridge A/RConn2 -- Vout_HBa/RConn1 -- DAB1_S20/RConn1
  Series RLC Branch/RConn1 -- Series RLC Branch7/LConn1 -- Voltage Measurement7/LConn1 -- Voltage Measurement/LConn2 -- D7/LConn1 -- D1/RConn1 -- D5/RConn1 -- Carga R con Filtro LC/LConn4 -- D4/LConn1 -- D3/RConn1 -- D2/LConn1
  Carga R con Filtro LC/LConn2 -- Subsystem8/LConn1 -- Subsystem7/RConn1
  Carga R con Filtro LC/LConn1 -- Subsystem5/LConn1 -- Subsystem1/RConn1
  Subsystem9/RConn1 -- Carga R con Filtro LC/LConn3 -- Subsystem10/LConn1
  D3/LConn1 -- Subsystem8/LConn2
  D7/RConn1 -- Subsystem1/LConn2
  D1/LConn1 -- Subsystem5/LConn2
  D4/RConn1 -- Subsystem9/LConn2
  D5/LConn1 -- Subsystem10/LConn2
  D2/RConn1 -- Subsystem7/LConn2
  Subsystem10/RConn1 -- Subsystem8/RConn1 -- Subsystem5/RConn1 -- Series RLC Branch7/RConn1 -- Voltage Measurement7/LConn2 -- DAB1_S15/RConn1 -- DAB1_S16/RConn1 -- Series RLC Branch16/RConn1 -- DAB1_S7/RConn1 -- DAB1_S8/RConn1 -- Series RLC Branch13/RConn1 -- Series RLC Branch14/RConn1 -- DAB1_S24/RConn1 -- DAB1_S23/RConn1

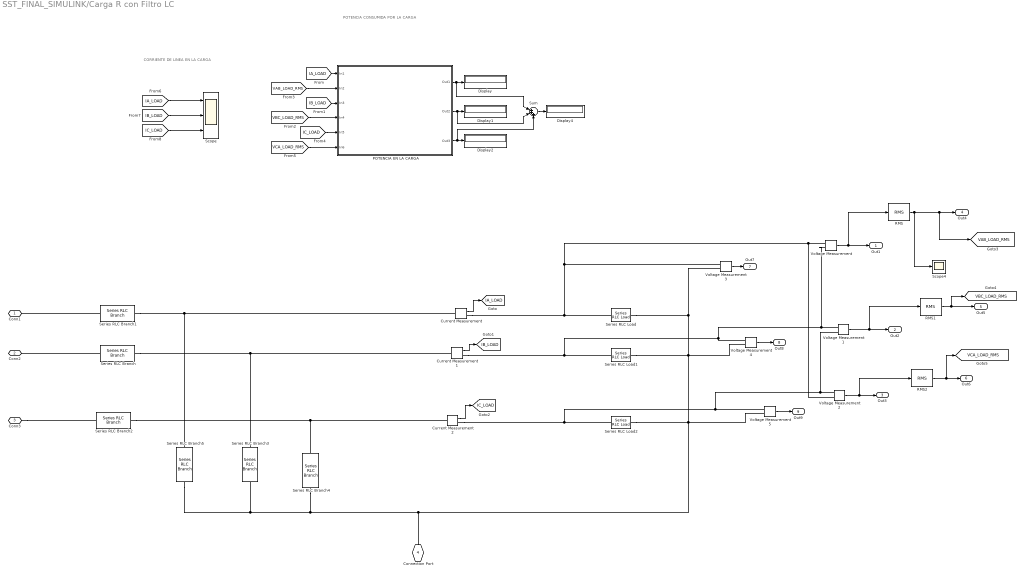
== system SST_FINAL_SIMULINK/Carga R con Filtro LC ==
  note: POTENCIA CONSUMIDA POR LA CARGA
  note: CORRIENTE DE LINEA EN LA CARGA
  Current Measurement : powerlib/Measurements/Current Measurement  PhasorSimulation=off  OutputType=Complex  PSBequivalent=0
  Current Measurement1 : powerlib/Measurements/Current Measurement  PhasorSimulation=off  OutputType=Complex  PSBequivalent=0
  Current Measurement2 : powerlib/Measurements/Current Measurement  PhasorSimulation=off  OutputType=Complex  PSBequivalent=0
  Display{,1..2,4} (4 alike) : Display
  "POTENCIA EN LA CARGA " : Subsystem
  RMS : powerlib_meascontrol/Measurements/RMS  TrueRMS=off  Freq=60  RMSInit=220  Ts=0
  RMS1 : powerlib_meascontrol/Measurements/RMS  TrueRMS=off  Freq=60  RMSInit=120  Ts=0
  RMS2 : powerlib_meascontrol/Measurements/RMS  TrueRMS=off  Freq=60  RMSInit=120  Ts=0
  Scope : Scope  NumInputPorts=3
  Scope4 : Scope
  Series RLC Branch : powerlib/Elements/Series RLC Branch  LConnTagsString=__new0  RConnTagsString=__new0  BranchType=L  Resistance=1  Inductance=L  SetiL0=off  InitialCurrent=0  Capacitance=1e-6  Setx0=off  InitialVoltage=0  Measurements=None
  Series RLC Branch1 : powerlib/Elements/Series RLC Branch  LConnTagsString=__new0  RConnTagsString=__new0  BranchType=L  Resistance=1  Inductance=L  SetiL0=off  InitialCurrent=0  Capacitance=1e-6  Setx0=off  InitialVoltage=0  Measurements=None
  Series RLC Branch2 : powerlib/Elements/Series RLC Branch  LConnTagsString=__new0  RConnTagsString=__new0  BranchType=L  Resistance=1  Inductance=L  SetiL0=off  InitialCurrent=0  Capacitance=1e-6  Setx0=off  InitialVoltage=0  Measurements=None
  Series RLC Branch3 : powerlib/Elements/Series RLC Branch  LConnTagsString=__new0  RConnTagsString=__new0  BranchType=C  Resistance=1  Inductance=L  SetiL0=off  InitialCurrent=0  Capacitance=ca  Setx0=off  InitialVoltage=0  Measurements=None
  Series RLC Branch4 : powerlib/Elements/Series RLC Branch  LConnTagsString=__new0  RConnTagsString=__new0  BranchType=C  Resistance=1  Inductance=ca  SetiL0=off  InitialCurrent=0  Capacitance=ca  Setx0=off  InitialVoltage=0  Measurements=None
  Series RLC Branch5 : powerlib/Elements/Series RLC Branch  LConnTagsString=__new0  RConnTagsString=__new0  BranchType=C  Resistance=1  Inductance=ca  SetiL0=off  InitialCurrent=0  Capacitance=ca  Setx0=off  InitialVoltage=0  Measurements=None
  Series RLC Load : powerlib/Elements/Series RLC Load  LConnTagsString=a  RConnTagsString=__new0  NominalVoltage=220/sqrt(3)  NominalFrequency=60  ActivePower=50e3/3  InductivePower=0  CapacitivePower=0  Setx0=off  InitialVoltage=0  SetiL0=off  InitialCurrent=0  Measurements=None  LoadType=constant Z
  Series RLC Load1 : powerlib/Elements/Series RLC Load  LConnTagsString=a  RConnTagsString=__new0  NominalVoltage=220/sqrt(3)  NominalFrequency=60  ActivePower=50e3/3  InductivePower=0  CapacitivePower=0  Setx0=off  InitialVoltage=0  SetiL0=off  InitialCurrent=0  Measurements=None  LoadType=constant Z
  Series RLC Load2 : powerlib/Elements/Series RLC Load  LConnTagsString=a  RConnTagsString=__new0  NominalVoltage=220/sqrt(3)  NominalFrequency=60  ActivePower=50e3/3  InductivePower=0  CapacitivePower=0  Setx0=off  InitialVoltage=0  SetiL0=off  InitialCurrent=0  Measurements=None  LoadType=constant Z
  Sum : Sum  Inputs=|+++
  Voltage Measurement{,1..5} (6 alike) : powerlib/Measurements/Voltage Measurement  PhasorSimulation=off  OutputType=Complex  PSBequivalent=0
  Conn1 : PMIOPort  Port=1  Side=Left
  Conn2 : PMIOPort  Port=2  Side=Left
  Conn3 : PMIOPort  Port=3  Side=Left
  Connection Port : PMIOPort  Tag=PMCPort  Port=4  Side=Left
  Out1 : Outport
  Out2 : Outport  Port=2
  Out3 : Outport  Port=3
  Out4 : Outport  Port=4
  Out5 : Outport  Port=5
  Out6 : Outport  Port=6
  Out7 : Outport  Port=7
  Out8 : Outport  Port=8
  Out9 : Outport  Port=9
  tag scope: IA_LOAD=global, IB_LOAD=global, IC_LOAD=global, VAB_LOAD_RMS=global, VBC_LOAD_RMS=global, VCA_LOAD_RMS=global
  wires:
  Voltage Measurement/1 -> RMS/1, Out1/1
  Voltage Measurement1/1 -> RMS1/1, Out2/1
  Voltage Measurement2/1 -> RMS2/1, Out3/1
  RMS/1 -> Scope4/1, [VAB_LOAD_RMS], Out4/1
  RMS1/1 -> [VBC_LOAD_RMS], Out5/1
  RMS2/1 -> [VCA_LOAD_RMS], Out6/1
  Current Measurement/1 -> [IA_LOAD]
  Current Measurement1/1 -> [IB_LOAD]
  Current Measurement2/1 -> [IC_LOAD]
  Voltage Measurement3/1 -> Out7/1
  Voltage Measurement4/1 -> Out8/1
  Voltage Measurement5/1 -> Out9/1
  [IA_LOAD] -> "POTENCIA EN LA CARGA "/1(In1)
  [VAB_LOAD_RMS] -> "POTENCIA EN LA CARGA "/2(In2)
  [IB_LOAD] -> "POTENCIA EN LA CARGA "/3(In3)
  [VBC_LOAD_RMS] -> "POTENCIA EN LA CARGA "/4(In4)
  [IC_LOAD] -> "POTENCIA EN LA CARGA "/5(In5)
  [VCA_LOAD_RMS] -> "POTENCIA EN LA CARGA "/6(In6)
  "POTENCIA EN LA CARGA "/1(Out1) -> Sum/1, Display/1
  "POTENCIA EN LA CARGA "/2(Out2) -> Sum/2, Display1/1
  "POTENCIA EN LA CARGA "/3(Out3) -> Sum/3, Display2/1
  [IA_LOAD] -> Scope/1
  [IB_LOAD] -> Scope/2
  [IC_LOAD] -> Scope/3
  Sum/1 -> Display4/1
  connections:
  Series RLC Branch5/RConn1 -- Series RLC Load2/RConn1 -- Series RLC Load1/RConn1 -- Series RLC Load/RConn1 -- Voltage Measurement3/LConn2 -- Voltage Measurement4/LConn2 -- Voltage Measurement5/LConn2 -- Connection Port/RConn1 -- Series RLC Branch4/RConn1 -- Series RLC Branch3/RConn1
  Series RLC Branch1/LConn1 -- Conn1/RConn1
  Series RLC Branch/LConn1 -- Conn2/RConn1
  Conn3/RConn1 -- Series RLC Branch2/LConn1
  Current Measurement/RConn1 -- Series RLC Load/LConn1 -- Voltage Measurement2/LConn2 -- Voltage Measurement/LConn1 -- Voltage Measurement3/LConn1
  Voltage Measurement/LConn2 -- Voltage Measurement1/LConn1 -- Series RLC Load1/LConn1 -- Current Measurement1/RConn1 -- Voltage Measurement4/LConn1
  Voltage Measurement1/LConn2 -- Voltage Measurement2/LConn1 -- Series RLC Load2/LConn1 -- Current Measurement2/RConn1 -- Voltage Measurement5/LConn1
  Series RLC Branch5/LConn1 -- Series RLC Branch1/RConn1 -- Current Measurement/LConn1
  Series RLC Branch2/RConn1 -- Series RLC Branch4/LConn1 -- Current Measurement2/LConn1
  Series RLC Branch3/LConn1 -- Series RLC Branch/RConn1 -- Current Measurement1/LConn1

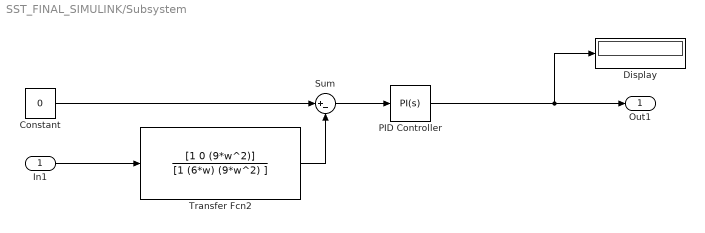
== system SST_FINAL_SIMULINK/Subsystem ==
  In1 : Inport
  Constant : Constant  Value=0  SampleTime=Ts
  Display : Display
  PID Controller : simulink/Continuous/PID Controller  Controller=PI  TimeDomain=Continuous-time  SampleTime=-1  IntegratorMethod=Forward Euler  FilterMethod=Forward Euler  Form=Parallel  UseFilter=on  ControllerParametersSource=internal  P=0  I=1  D=0.1  N=100  InitialConditionSource=internal  InitialConditionForIntegrator=0  InitialConditionForFilter=0  ExternalReset=none  LimitOutput=off  UpperSaturationLimit=inf  LowerSaturationLimit=-inf  LinearizeAsGain=on  AntiWindupMode=none  Kb=1  TrackingMode=off  Kt=1  PParamMin=[]  PParamMax=[]  IParamMin=[]  IParamMax=[]  DParamMin=[]  DParamMax=[]  NParamMin=[]  NParamMax=[]  KbParamMin=[]  KbParamMax=[]  KtParamMin=[]  KtParamMax=[]  POutMin=[]  POutMax=[]  IOutMin=[]  IOutMax=[]  DOutMin=[]  DOutMax=[]  NOutMin=[]  NOutMax=[]  KbOutMin=[]  KbOutMax=[]  KtOutMin=[]  KtOutMax=[]  IntegratorOutMin=[]  IntegratorOutMax=[]  FilterOutMin=[]  FilterOutMax=[]  SumOutMin=[]  SumOutMax=[]  SumI1OutMin=[]  SumI1OutMax=[]  SumI2OutMin=[]  SumI2OutMax=[]  SumI3OutMin=[]  SumI3OutMax=[]  SumDOutMin=[]  SumDOutMax=[]  SaturationOutMin=[]  SaturationOutMax=[]  IntegratorContinuousStateAttributes=''  IntegratorStateMustResolveToSignalObject=off  IntegratorRTWStateStorageClass=Auto  FilterContinuousStateAttributes=''  FilterStateMustResolveToSignalObject=off  FilterRTWStateStorageClass=Auto  DifferentiatorICPrevScaledInput=0  DifferentiatorOutMin=[]  DifferentiatorOutMax=[]  InitialConditionSetting=State (most efficient)  FilterDiffOutCoefMin=[]  FilterDiffOutCoefMax=[]  SumDenOutMin=[]  SumDenOutMax=[]  SumNumOutMin=[]  SumNumOutMax=[]  ReciprocalOutMin=[]  ReciprocalOutMax=[]  DivideOutMin=[]  DivideOutMax=[]  TunerSelectOption=Transfer Function Based (PID Tuner App)
  Sum : Sum  Inputs=|+-
  Transfer Fcn2 : TransferFcn  Numerator=[1 0 (9*w^2)]  Denominator=[1 (6*w) (9*w^2) ]
  Out1 : Outport
  wires:
  In1/1 -> Transfer Fcn2/1
  Constant/1 -> Sum/1
  Sum/1 -> PID Controller/1
  Transfer Fcn2/1 -> Sum/2
  PID Controller/1 -> Out1/1, Display/1

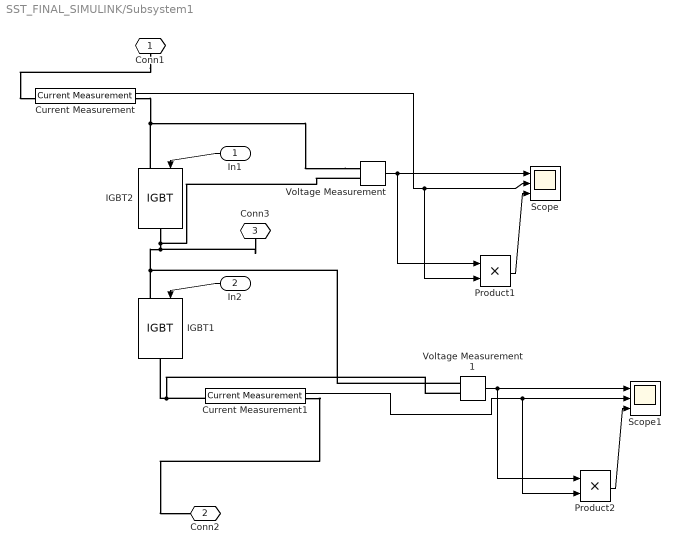
== system SST_FINAL_SIMULINK/Subsystem1 ==
  In1 : Inport
  In2 : Inport  Port=2
  Current Measurement : powerlib/Measurements/Current Measurement  PhasorSimulation=off  OutputType=Complex  PSBequivalent=0
  Current Measurement1 : powerlib/Measurements/Current Measurement  PhasorSimulation=off  OutputType=Complex  PSBequivalent=0
  IGBT1 : powerlib/Power Electronics/IGBT  Ron=0.000000001  Lon=0  Vf=0  Tf=1e-6  Tt=2e-6  IC=0  Rs=1e5  Cs=inf  Measurements=off
  IGBT2 : powerlib/Power Electronics/IGBT  Ron=0.000000001  Lon=0  Vf=0  Tf=1e-6  Tt=2e-6  IC=0  Rs=inf  Cs=inf  Measurements=off
  Product1 : Product
  Product2 : Product
  Scope : Scope  NumInputPorts=3
  Scope1 : Scope  NumInputPorts=3
  Voltage Measurement : powerlib/Measurements/Voltage Measurement  PhasorSimulation=off  OutputType=Complex  PSBequivalent=0
  Voltage Measurement1 : powerlib/Measurements/Voltage Measurement  PhasorSimulation=off  OutputType=Complex  PSBequivalent=0
  Conn1 : PMIOPort  Port=1  Side=Left
  Conn2 : PMIOPort  Port=2  Side=Right
  Conn3 : PMIOPort  Port=3  Side=Left
  wires:
  In2/1 -> IGBT1/1
  In1/1 -> IGBT2/1
  Voltage Measurement/1 -> Product1/1, Scope/1
  Current Measurement/1 -> Product1/2, Scope/2
  Product1/1 -> Scope/3
  Product2/1 -> Scope1/3
  Voltage Measurement1/1 -> Scope1/1, Product2/1
  Current Measurement1/1 -> Product2/2, Scope1/2
  connections:
  Voltage Measurement/LConn1 -- IGBT2/LConn1 -- Current Measurement/RConn1
  Conn3/RConn1 -- Voltage Measurement1/LConn1 -- IGBT1/LConn1 -- IGBT2/RConn1 -- Voltage Measurement/LConn2
  Conn1/RConn1 -- Current Measurement/LConn1
  Current Measurement1/LConn1 -- Voltage Measurement1/LConn2 -- IGBT1/RConn1
  Current Measurement1/RConn1 -- Conn2/RConn1

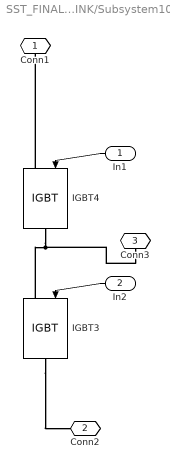
== system SST_FINAL_SIMULINK/Subsystem10 ==
  In1 : Inport
  In2 : Inport  Port=2
  IGBT3 : powerlib/Power Electronics/IGBT  Ron=0.000000001  Lon=0  Vf=0  Tf=1e-6  Tt=2e-6  IC=0  Rs=1e5  Cs=inf  Measurements=off
  IGBT4 : powerlib/Power Electronics/IGBT  Ron=0.000000001  Lon=0  Vf=0  Tf=1e-6  Tt=2e-6  IC=0  Rs=inf  Cs=inf  Measurements=off
  Conn1 : PMIOPort  Port=1  Side=Left
  Conn2 : PMIOPort  Port=2  Side=Right
  Conn3 : PMIOPort  Port=3  Side=Left
  wires:
  In1/1 -> IGBT4/1
  In2/1 -> IGBT3/1
  connections:
  Conn3/RConn1 -- IGBT4/RConn1 -- IGBT3/LConn1
  IGBT3/RConn1 -- Conn2/RConn1
  IGBT4/LConn1 -- Conn1/RConn1

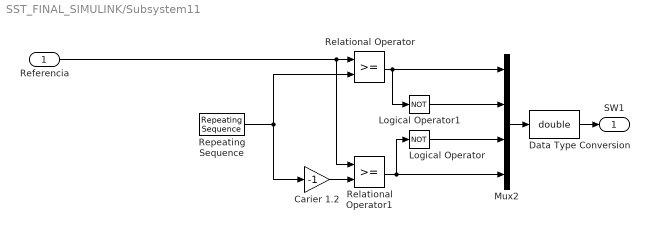
== system SST_FINAL_SIMULINK/Subsystem11 ==
  Referencia : Inport
  Carier 1.2 : Gain  Gain=-1
  Data Type Conversion : DataTypeConversion  OutDataTypeStr=double
  Logical Operator : Logic  Operator=NOT  IconShape=distinctive  AllPortsSameDT=off  OutDataTypeStr=boolean
  Logical Operator1 : Logic  Operator=NOT  IconShape=distinctive  AllPortsSameDT=off  OutDataTypeStr=boolean
  Mux2 : Mux
  Relational Operator : RelationalOperator  OutDataTypeStr=boolean  RndMeth=Simplest
  Relational Operator1 : RelationalOperator  OutDataTypeStr=boolean  RndMeth=Simplest
  Repeating Sequence : simulink/Sources/Repeating Sequence  rep_seq_t=[0 0.5 1]/Fsw_HB  rep_seq_y=[0 1 0]
  SW1 : Outport
  wires:
  Referencia/1 -> Relational Operator/1, Relational Operator1/1
  Repeating Sequence/1 -> Carier 1.2/1, Relational Operator/2
  Logical Operator1/1 -> Mux2/2
  Data Type Conversion/1 -> SW1/1
  Mux2/1 -> Data Type Conversion/1
  Logical Operator/1 -> Mux2/3
  Relational Operator/1 -> Mux2/1, Logical Operator1/1
  Carier 1.2/1 -> Relational Operator1/2
  Relational Operator1/1 -> Mux2/4, Logical Operator/1

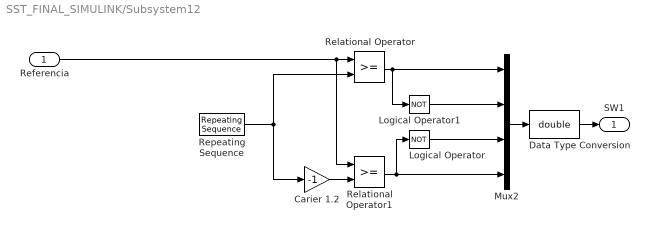
== system SST_FINAL_SIMULINK/Subsystem12 ==
  Referencia : Inport
  Carier 1.2 : Gain  Gain=-1
  Data Type Conversion : DataTypeConversion  OutDataTypeStr=double
  Logical Operator : Logic  Operator=NOT  IconShape=distinctive  AllPortsSameDT=off  OutDataTypeStr=boolean
  Logical Operator1 : Logic  Operator=NOT  IconShape=distinctive  AllPortsSameDT=off  OutDataTypeStr=boolean
  Mux2 : Mux
  Relational Operator : RelationalOperator  OutDataTypeStr=boolean  RndMeth=Simplest
  Relational Operator1 : RelationalOperator  OutDataTypeStr=boolean  RndMeth=Simplest
  Repeating Sequence : simulink/Sources/Repeating Sequence  rep_seq_t=[0 0.5 1]/Fsw_HB  rep_seq_y=[0 1 0]
  SW1 : Outport
  wires:
  Relational Operator1/1 -> Logical Operator/1, Mux2/4
  Carier 1.2/1 -> Relational Operator1/2
  Relational Operator/1 -> Logical Operator1/1, Mux2/1
  Logical Operator/1 -> Mux2/3
  Mux2/1 -> Data Type Conversion/1
  Data Type Conversion/1 -> SW1/1
  Logical Operator1/1 -> Mux2/2
  Repeating Sequence/1 -> Relational Operator/2, Carier 1.2/1
  Referencia/1 -> Relational Operator1/1, Relational Operator/1

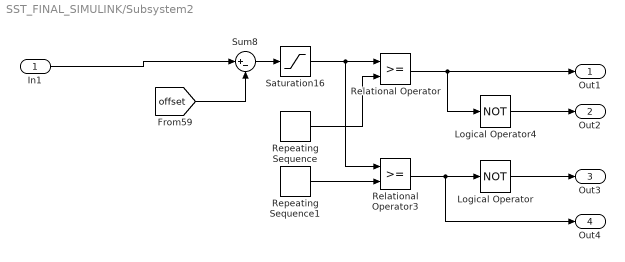
== system SST_FINAL_SIMULINK/Subsystem2 ==
  In1 : Inport
  Logical Operator : Logic  Operator=NOT  AllPortsSameDT=off  OutDataTypeStr=boolean
  Logical Operator4 : Logic  Operator=NOT  AllPortsSameDT=off  OutDataTypeStr=boolean
  Relational Operator : RelationalOperator  ZeroCross=off  RndMeth=Nearest
  Relational Operator3 : RelationalOperator  ZeroCross=off  RndMeth=Nearest
  Repeating Sequence : simulink/Sources/Repeating Sequence  rep_seq_t=[0 0.5/Fsw_NPC 1/Fsw_NPC]  rep_seq_y=[ 0 1 0 ]
  Repeating Sequence1 : simulink/Sources/Repeating Sequence  rep_seq_t=[0 0.5/Fsw_NPC 1/Fsw_NPC]  rep_seq_y=[-1 0 -1]
  Saturation16 : Saturate  UpperLimit=m  LowerLimit=-m  ZeroCross=off
  Sum8 : Sum  Inputs=|+-
  Out1 : Outport
  Out2 : Outport  Port=2
  Out3 : Outport  Port=3
  Out4 : Outport  Port=4
  wires:
  In1/1 -> Sum8/1
  Relational Operator3/1 -> Out4/1, Logical Operator/1
  [offset] -> Sum8/2
  Relational Operator/1 -> Out1/1, Logical Operator4/1
  Repeating Sequence/1 -> Relational Operator/2
  Sum8/1 -> Saturation16/1
  Logical Operator4/1 -> Out2/1
  Logical Operator/1 -> Out3/1
  Repeating Sequence1/1 -> Relational Operator3/2
  Saturation16/1 -> Relational Operator3/1, Relational Operator/1
